simulink model "quadcopter"  (R2025b)
settings: Solver=VariableStepAuto  StartTime=0.0  StopTime=10.0  RelTol=1e-3
undefined symbols (not defined in the file or in its folder): p_init, phi_init, psi_init, q_init, r_init, theta_init, u_init, v_init, w_init, x_init, y_init, z_init
settings Model: Creator=deepa  LastModifiedBy=deepa

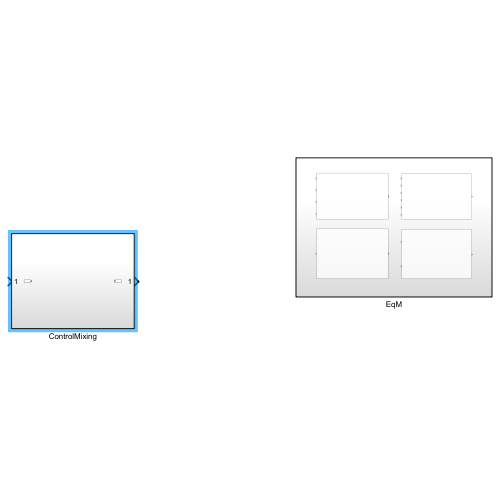
[thumbnail: Simulink's stored preview of the top-level diagram]
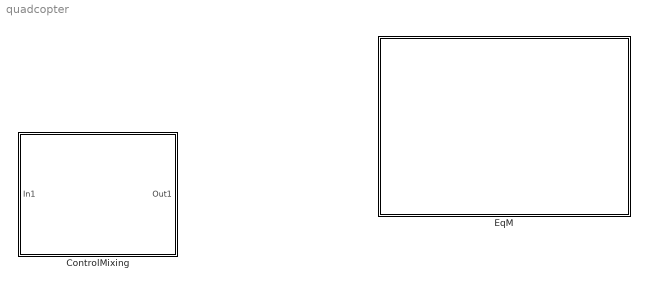
== system quadcopter ==
  ControlMixing : Subsystem
  EqM : Subsystem

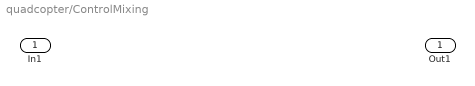
== system quadcopter/ControlMixing ==
  In1 : Inport
  Out1 : Outport

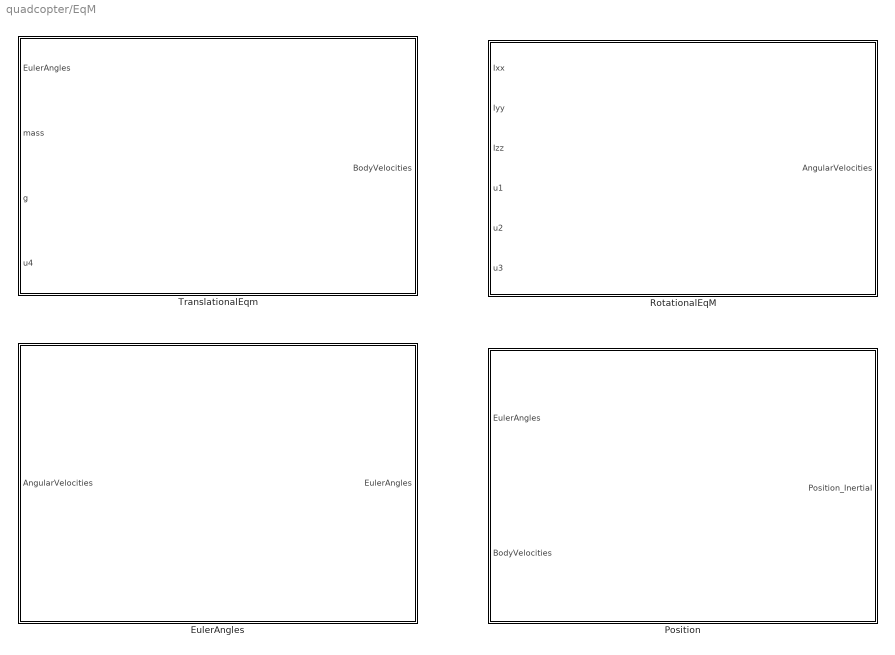
== system quadcopter/EqM ==
  EulerAngles : Subsystem
  Position : Subsystem
  RotationalEqM : Subsystem
  TranslationalEqm : Subsystem

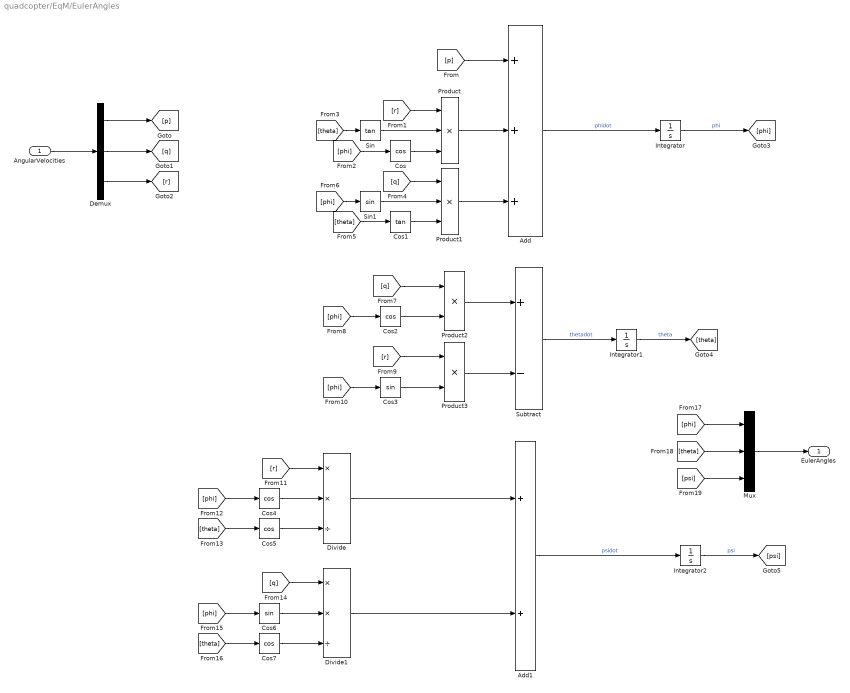
== system quadcopter/EqM/EulerAngles ==
  AngularVelocities : Inport
  Add : Sum  Inputs=+++
  Add1 : Sum
  Cos{,2,4..5,7} (5 alike) : Trigonometry  Operator=cos
  Cos1 : Trigonometry  Operator=tan
  Cos3 : Trigonometry
  Cos6 : Trigonometry
  Demux : Demux  Outputs=3
  Divide : Product  Inputs=**/
  Divide1 : Product  Inputs=**/
  Integrator : Integrator  InitialCondition=phi_init  ContinuousStateAttributes='phi'
  Integrator1 : Integrator  InitialCondition=theta_init  ContinuousStateAttributes='theta'
  Integrator2 : Integrator  InitialCondition=psi_init  ContinuousStateAttributes='psi'
  Mux : Mux  Inputs=3
  Product : Product  Inputs=3
  Product1 : Product  Inputs=3
  Product2 : Product
  Product3 : Product
  Sin : Trigonometry  Operator=tan
  Sin1 : Trigonometry
  Subtract : Sum  Inputs=+-
  EulerAngles : Outport
  wires:
  AngularVelocities/1 -> Demux/1
  Demux/1 -> [p]
  Demux/2 -> [q]
  Demux/3 -> [r]
  Integrator/1 -> [phi]  "phi"
  Integrator1/1 -> [theta]  "theta"
  Integrator2/1 -> [psi]  "psi"
  [phi] -> Cos/1
  [theta] -> Sin/1
  [r] -> Product/1
  Sin/1 -> Product/2
  Cos/1 -> Product/3
  [theta] -> Cos1/1
  Sin1/1 -> Product1/2
  [q] -> Product1/1
  Cos1/1 -> Product1/3
  [phi] -> Sin1/1
  [p] -> Add/1
  Product/1 -> Add/2
  Product1/1 -> Add/3
  Add/1 -> Integrator/1  "phidot"
  [phi] -> Cos2/1
  [q] -> Product2/1
  Cos2/1 -> Product2/2
  [r] -> Product3/1
  Cos3/1 -> Product3/2
  [phi] -> Cos3/1
  Product2/1 -> Subtract/1
  Product3/1 -> Subtract/2
  Subtract/1 -> Integrator1/1  "thetadot"
  [phi] -> Cos4/1
  [theta] -> Cos5/1
  [r] -> Divide/1
  Cos4/1 -> Divide/2
  Cos5/1 -> Divide/3
  [theta] -> Cos7/1
  Cos7/1 -> Divide1/3
  Cos6/1 -> Divide1/2
  [q] -> Divide1/1
  [phi] -> Cos6/1
  Divide1/1 -> Add1/2
  Divide/1 -> Add1/1
  Add1/1 -> Integrator2/1  "psidot"
  [phi] -> Mux/1
  [theta] -> Mux/2
  [psi] -> Mux/3
  Mux/1 -> EulerAngles/1

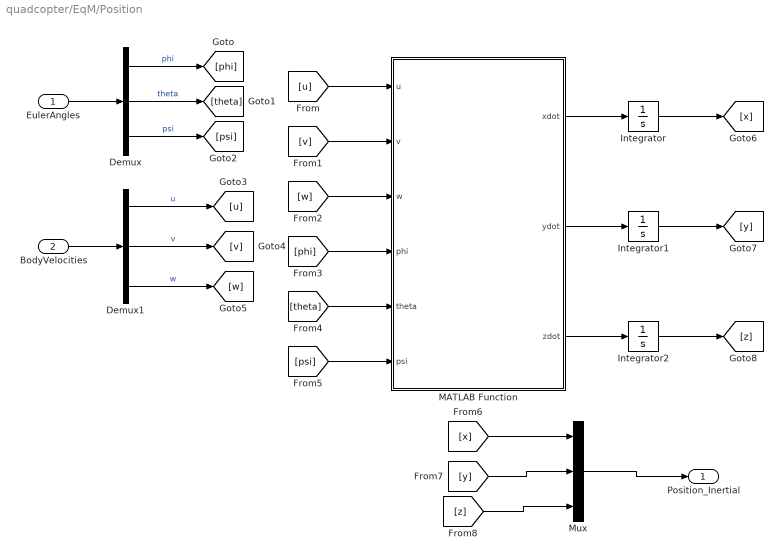
== system quadcopter/EqM/Position ==
  EulerAngles : Inport
  BodyVelocities : Inport  Port=2
  Demux : Demux  Outputs=3
  Demux1 : Demux  Outputs=3
  Integrator : Integrator  InitialCondition=x_init  ContinuousStateAttributes='x'
  Integrator1 : Integrator  InitialCondition=y_init  ContinuousStateAttributes='y'
  Integrator2 : Integrator  InitialCondition=z_init  ContinuousStateAttributes='z'
  MATLAB Function : MATLAB Function  TreatAsAtomicUnit=on
  Mux : Mux  Inputs=3
  Position_Inertial : Outport
  wires:
  EulerAngles/1 -> Demux/1
  BodyVelocities/1 -> Demux1/1
  Demux/1 -> [phi]  "phi"
  Demux/2 -> [theta]  "theta"
  Demux/3 -> [psi]  "psi"
  Demux1/1 -> [u]  "u"
  Demux1/2 -> [v]  "v"
  Demux1/3 -> [w]  "w"
  [u] -> MATLAB Function/1(u)
  [v] -> MATLAB Function/2(v)
  [w] -> MATLAB Function/3(w)
  [phi] -> MATLAB Function/4(phi)
  [theta] -> MATLAB Function/5(theta)
  [psi] -> MATLAB Function/6(psi)
  MATLAB Function/1(xdot) -> Integrator/1
  MATLAB Function/2(ydot) -> Integrator1/1
  MATLAB Function/3(zdot) -> Integrator2/1
  Integrator/1 -> [x]
  Integrator1/1 -> [y]
  Integrator2/1 -> [z]
  [x] -> Mux/1
  [y] -> Mux/2
  [z] -> Mux/3
  Mux/1 -> Position_Inertial/1

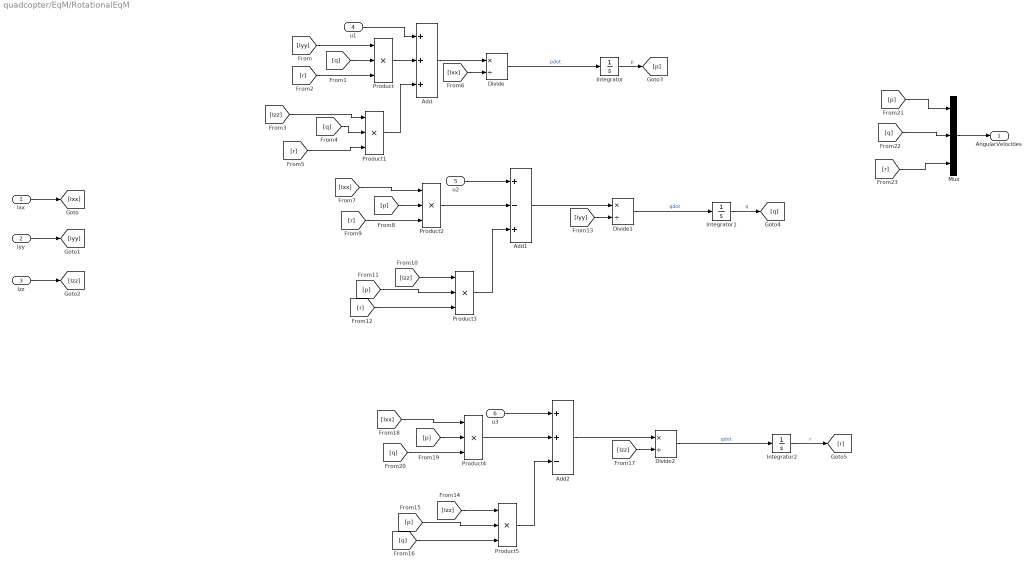
== system quadcopter/EqM/RotationalEqM ==
  Ixx : Inport
  Iyy : Inport  Port=2
  Izz : Inport  Port=3
  u1 : Inport  Port=4
  u2 : Inport  Port=5
  u3 : Inport  Port=6
  Add : Sum  Inputs=+++
  Add1 : Sum  Inputs=+-+
  Add2 : Sum  Inputs=++-
  Divide : Product  Inputs=*/
  Divide1 : Product  Inputs=*/
  Divide2 : Product  Inputs=*/
  Integrator : Integrator  InitialCondition=p_init  ContinuousStateAttributes='p'
  Integrator1 : Integrator  InitialCondition=q_init  ContinuousStateAttributes='q'
  Integrator2 : Integrator  InitialCondition=r_init  ContinuousStateAttributes='r'
  Mux : Mux  Inputs=3
  Product{,1..5} (6 alike) : Product  Inputs=3
  AngularVelocities : Outport
  wires:
  Ixx/1 -> [Ixx]
  Iyy/1 -> [Iyy]
  Izz/1 -> [Izz]
  Integrator/1 -> [p]  "p"
  Divide1/1 -> Integrator1/1  "qdot"
  Integrator1/1 -> [q]  "q"
  Integrator2/1 -> [r]  "r"
  [Iyy] -> Product/1
  [q] -> Product/2
  [r] -> Product/3
  Product/1 -> Add/2
  u1/1 -> Add/1
  [Izz] -> Product1/1
  [r] -> Product1/3
  [q] -> Product1/2
  Product1/1 -> Add/3
  Divide/1 -> Integrator/1  "pdot"
  Add/1 -> Divide/1
  [Ixx] -> Divide/2
  u2/1 -> Add1/1
  [Ixx] -> Product2/1
  Product2/1 -> Add1/2
  Product3/1 -> Add1/3
  [p] -> Product3/2
  [r] -> Product3/3
  [r] -> Product2/3
  [p] -> Product2/2
  Add1/1 -> Divide1/1
  [Iyy] -> Divide1/2
  [Izz] -> Product3/1
  u3/1 -> Add2/1
  [Izz] -> Divide2/2
  [p] -> Product5/2
  [q] -> Product4/3
  [p] -> Product4/2
  [Izz] -> Product5/1
  Product5/1 -> Add2/3
  Product4/1 -> Add2/2
  [q] -> Product5/3
  Add2/1 -> Divide2/1
  [Ixx] -> Product4/1
  Divide2/1 -> Integrator2/1  "qdot"
  [r] -> Mux/3
  [q] -> Mux/2
  [p] -> Mux/1
  Mux/1 -> AngularVelocities/1

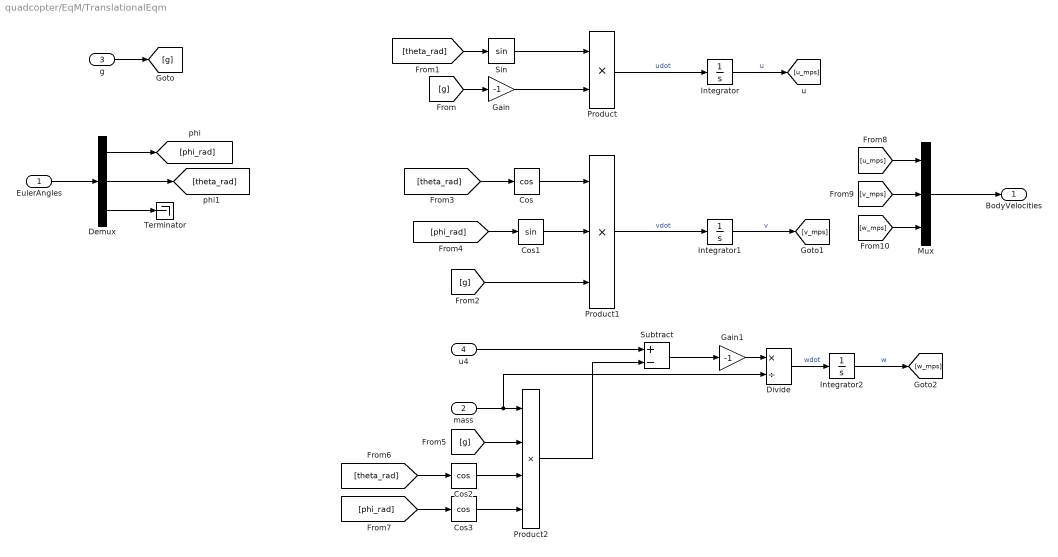
== system quadcopter/EqM/TranslationalEqm ==
  EulerAngles : Inport
  mass : Inport  Port=2
  g : Inport  Port=3
  u4 : Inport  Port=4
  Cos : Trigonometry  Operator=cos
  Cos1 : Trigonometry
  Cos2 : Trigonometry  Operator=cos
  Cos3 : Trigonometry  Operator=cos
  Demux : Demux  Outputs=3
  Divide : Product  Inputs=*/
  Gain : Gain  Gain=-1
  Gain1 : Gain  Gain=-1
  Integrator : Integrator  InitialCondition=u_init  ContinuousStateAttributes='u'
  Integrator1 : Integrator  InitialCondition=v_init  ContinuousStateAttributes='v'
  Integrator2 : Integrator  InitialCondition=w_init  ContinuousStateAttributes='w'
  Mux : Mux  Inputs=3
  Product : Product
  Product1 : Product  Inputs=3
  Product2 : Product  Inputs=4
  Sin : Trigonometry
  Subtract : Sum  Inputs=+-
  Terminator : Terminator
  BodyVelocities : Outport
  wires:
  [g] -> Product2/2
  [theta_rad] -> Cos/1
  Sin/1 -> Product/1
  Subtract/1 -> Gain1/1
  [g] -> Gain/1
  Gain1/1 -> Divide/1
  [phi_rad] -> Cos1/1
  u4/1 -> Subtract/1
  Demux/2 -> [theta_rad]
  Demux/3 -> Terminator/1
  [theta_rad] -> Sin/1
  Demux/1 -> [phi_rad]
  EulerAngles/1 -> Demux/1
  Cos2/1 -> Product2/3
  [phi_rad] -> Cos3/1
  Cos3/1 -> Product2/4
  Integrator/1 -> [u_mps]  "u"
  [theta_rad] -> Cos2/1
  Cos/1 -> Product1/1
  Integrator1/1 -> [v_mps]  "v"
  Product1/1 -> Integrator1/1  "vdot"
  g/1 -> [g]
  mass/1 -> Divide/2, Product2/1
  Product/1 -> Integrator/1  "udot"
  Gain/1 -> Product/2
  Divide/1 -> Integrator2/1  "wdot"
  Cos1/1 -> Product1/2
  [g] -> Product1/3
  Product2/1 -> Subtract/2
  Integrator2/1 -> [w_mps]  "w"
  [u_mps] -> Mux/1
  [v_mps] -> Mux/2
  [w_mps] -> Mux/3
  Mux/1 -> BodyVelocities/1

== matlab function quadcopter/EqM/Position/MATLAB Function ==
  data: u input; xdot output; v input; w input; phi input; theta input; psi input; ydot output; zdot output
function [xdot, ydot, zdot] = Pos(u, v, w, phi ,theta, psi)

xdot = w*(sin(phi)*sin(psi) + cos(phi)*cos(psi)*sin(theta)) - v*(cos(phi)*sin(psi) - cos(psi)*sin(phi)*sin(theta)) + u*cos(psi)*cos(theta);
ydot = v*(cos(phi)*cos(psi) + sin(phi)*sin(psi)*sin(theta)) - w*(cos(psi)*sin(phi) - cos(phi)*sin(psi)*sin(theta)) + u*cos(theta)*sin(psi);
zdot = w*cos(phi)*cos(theta) - u*sin(theta) + v*cos(theta)*sin(phi);

end
